simulink model "tp3_controleur"  (R2023b)
settings: Solver=ode45  StartTime=0.0  StopTime=tf  RelTol=1e-3
values from neighbouring files (symbols this model uses):
  ue = 0    [parameters.m]
  x0 = [0 0 0 0]    [parameters.m]
  xe = [0 0 0 0]    [parameters.m]
undefined symbols (not defined in the file or in its folder): K
settings Model: Creator=cycy  LastModifiedBy=cycy

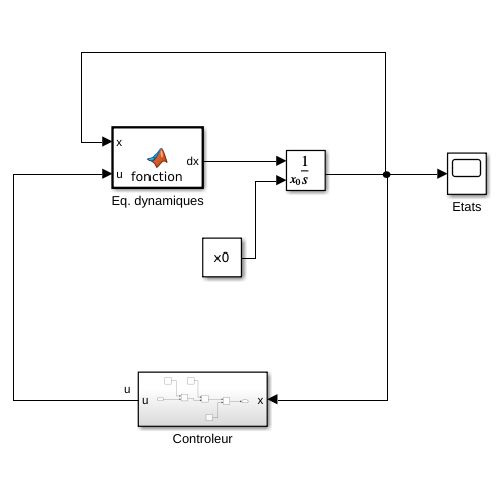
[thumbnail: Simulink's stored preview of the top-level diagram]
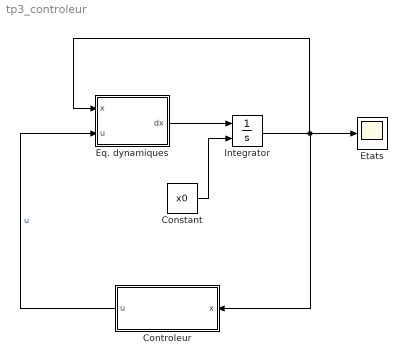
== system tp3_controleur ==
  Constant : Constant  Value=x0
  Controleur : Subsystem
  Eq. dynamiques : MATLAB Function  TreatAsAtomicUnit=on
  Etats : Scope
  Integrator : Integrator  InitialConditionSource=external
  wires:
  Constant/1 -> Integrator/2
  Controleur/1(u) -> Eq. dynamiques/2(u)  "u"
  Eq. dynamiques/1(dx) -> Integrator/1
  Integrator/1 -> Eq. dynamiques/1(x), Controleur/1(x), Etats/1

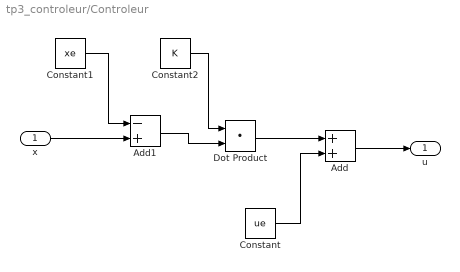
== system tp3_controleur/Controleur ==
  x : Inport
  Add : Sum
  Add1 : Sum  Inputs=-+
  Constant : Constant  Value=ue
  Constant1 : Constant  Value=xe
  Constant2 : Constant  Value=K
  Dot Product : DotProduct  OutDataTypeStr=Inherit: Inherit via internal rule
  u : Outport
  wires:
  Constant/1 -> Add/2
  x/1 -> Add1/2
  Constant1/1 -> Add1/1
  Dot Product/1 -> Add/1
  Add1/1 -> Dot Product/2
  Constant2/1 -> Dot Product/1
  Add/1 -> u/1

== matlab function tp3_controleur/Eq. dynamiques ==
  data: x input; u input; dx output
function dx   = fonction( x, u)
%   Dynamic equations of motion of the segway on an axis.
%   Inputs: - x = [theta psi dtheta dpsi]
%               theta: average angle of the wheels      [rad]
%               psi: body pitch angle                   [rad]
%               dtheta: average velocity of the wheels  [rad/s]
%               dpsi: body pitch velocity               [rad/s]
%          - u: DC motor voltage (same value for both motors) [V]

    % State
    psi = x(2);
    dtheta = x(3);
    dpsi = x(4);

    % Parameters
    
    g = 9.81;           % gravity acceleration [m/sec^2]
    m = 0.03;           % wheel weight [kg]
    R = 0.04;           % wheel radius [m]
    Jw = m*R^2/2;       % wheel inertia moment [kg*m^2]
    M = 0.6;            % body weight [kg]
    H = 0.144;          % body height [m]
    L = H/2;            % distance of the center of mass from the wheel axle [m]
    Jpsi = M*L^2/3;     % body pitch inertia [kgm^2]
    Jm = 1e-5;          % DC motor inertia moment [kgm^2]
    Rm = 6.69;          % DC motor resistance [Ohm]
    Kb = 0.468;         % DC motor back EMF constant [Vsec/rad]
    Kt = 0.317;         % DC motor torque constant [Nm/A]
    n = 1;              % gear ratio
    fm = 0.0022;        % friction coefficient between body and DC motor
    fw = 0;             % friction coefficient between wheel and floor
    
    % Equations of motion
    c1 = (2*m+M)*R^2 + 2*Jw + 2*n^2*Jm;
    c2 = M*L*R*cos(psi) - 2*n^2*Jm;
    c3 = -M*L*R*dpsi^2*sin(psi);
    c4 = M*L^2 + Jpsi + 2*n^2*Jm;
    c5 = -M*g*L*sin(psi);

    alpha = Kt/Rm;
    beta = Kt*Kb/Rm + fm;

    Ftheta = alpha*(2*u) - 2*(beta+fw)*dtheta + 2*beta*dpsi;
    Fpsi = -alpha*(2*u) + 2*beta*dtheta - 2*beta*dpsi;

    ddtheta = (c4*c3 - c2*c5 + c4*Ftheta - c2*Fpsi)/(c4*c1 - c2^2);
    ddpsi = (Fpsi- c2*ddtheta - c5)/c4;
    dx = [dtheta dpsi ddtheta ddpsi]';

end
